simulink model "Schimmel_Evan_lab_1_model"  (R2021a)
settings: Solver=VariableStepAuto  StartTime=0.0  StopTime=tf  MaxStep=maxstep  RelTol=tol  AbsTol=tol
values from neighbouring files (symbols this model uses):
  c = cLab    [Schimmel_Evan_lab_1_script.m]
  Fin = 4    [Schimmel_Evan_lab_1_script.m]
  k = kLab    [Schimmel_Evan_lab_1_script.m]
  m = mLab    [Schimmel_Evan_lab_1_script.m]
  v0 = 0    [Schimmel_Evan_lab_1_script.m]
  x0 = 0    [Schimmel_Evan_lab_1_script.m]
settings Model: Creator=schimmer  LastModifiedBy=schimmer
settings SolverCC: AlgebraicLoopSolver=TrustRegion
settings DataIOCC: SaveOutput=off  SignalLogging=off  DSMLogging=off  SaveTime=off  ReturnWorkspaceOutputs=off
settings DebuggingCC: SFMachineParentedDataDiag=warning

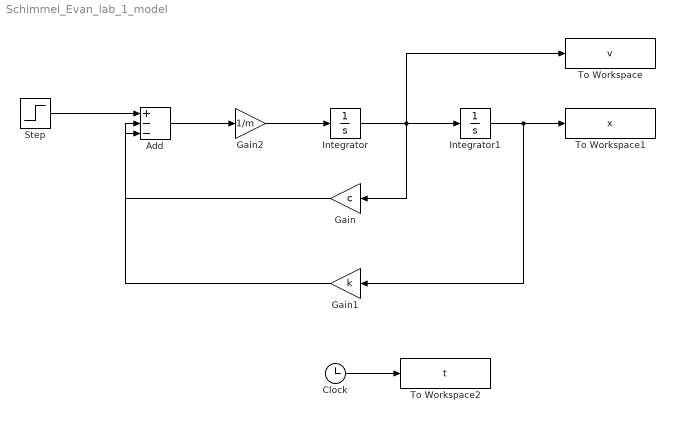
== system Schimmel_Evan_lab_1_model ==
  Add : Sum  Inputs=+--
  Clock : Clock
  Gain : Gain  Gain=c
  Gain1 : Gain  Gain=k
  Gain2 : Gain  Gain=1/m
  Integrator : Integrator  InitialCondition=v0
  Integrator1 : Integrator  InitialCondition=x0
  Step : Step  Time=0  After=Fin  SampleTime=0
  To Workspace : ToWorkspace  VariableName=v  SampleTime=-1
  To Workspace1 : ToWorkspace  VariableName=x  SampleTime=-1
  To Workspace2 : ToWorkspace  VariableName=t  SampleTime=-1
  wires:
  Integrator/1 -> To Workspace/1, Integrator1/1, Gain/1
  Integrator1/1 -> Gain1/1, To Workspace1/1
  Add/1 -> Gain2/1
  Gain2/1 -> Integrator/1
  Gain1/1 -> Add/2
  Gain/1 -> Add/3
  Step/1 -> Add/1
  Clock/1 -> To Workspace2/1
